simulink model "model"  (R2023b)
settings: Solver=FixedStepAuto  StartTime=0.0  StopTime=10.0  FixedStep=1e-3  RelTol=1e-3
InitFcn:
  | model_init
StopFcn:
  | animation;
values from neighbouring files (symbols this model uses):
  g = 9.81    [model_init.m]
  K = lqr(sys, Q, R)    [generate_controller.m]
  l = 1    [model_init.m]
  m = 0.5    [model_init.m]
  M = 1    [model_init.m]
  theta = out.simout.theta.Data    [animation.m]    (also in model_init.m = 0)
  theta_dot = 0    [model_init.m]
  x = out.simout.x.Data    [animation.m]    (also in model_init.m = 0)
  x_dot = 0    [model_init.m]
settings Model: Creator=zbyss  LastModifiedBy=zbyss

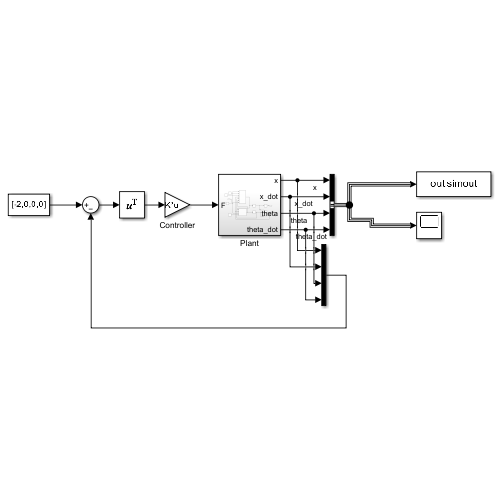
[thumbnail: Simulink's stored preview of the top-level diagram]
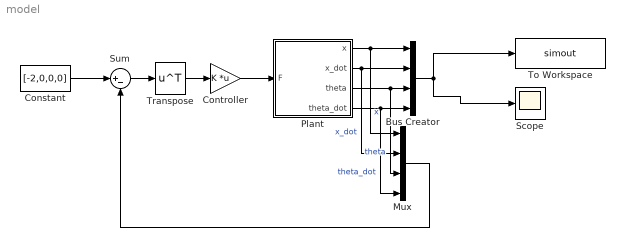
== system model ==
  Bus Creator : BusCreator  Inputs=4
  Constant : Constant  Value=[-2,0,0,0]
  Controller : Gain  Gain=K  Multiplication=Matrix(K*u)
  Mux : Mux
  Plant : Subsystem
  Scope : Scope
  Sum : Sum  Inputs=|+-
  To Workspace : ToWorkspace  VariableName=simout  SaveFormat=Timeseries  SampleTime=-1
  Transpose : Math  Operator=transpose
  wires:
  Plant/1(x) -> Bus Creator/1, Mux/1  "x"
  Plant/2(x_dot) -> Bus Creator/2, Mux/2  "x_dot"
  Plant/3(theta) -> Mux/3, Bus Creator/3  "theta"
  Plant/4(theta_dot) -> Mux/4, Bus Creator/4  "theta_dot"
  Bus Creator/1 -> To Workspace/1, Scope/1
  Controller/1 -> Plant/1(F)
  Transpose/1 -> Controller/1
  Sum/1 -> Transpose/1
  Mux/1 -> Sum/2
  Constant/1 -> Sum/1

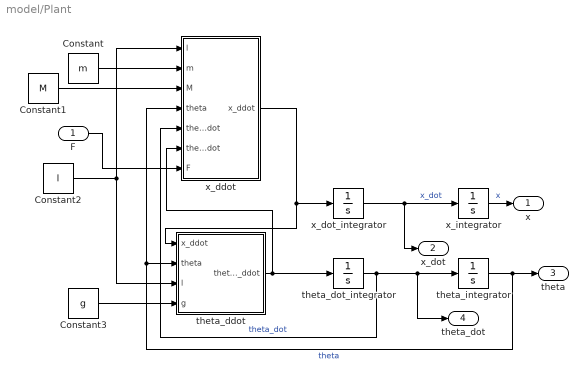
== system model/Plant ==
  F : Inport
  Constant : Constant  Value=m
  Constant1 : Constant  Value=M
  Constant2 : Constant  Value=l
  Constant3 : Constant  Value=g
  theta_ddot : Subsystem
  theta_dot_integrator : Integrator  InitialCondition=theta_dot
  theta_integrator : Integrator  InitialCondition=theta
  x_ddot : Subsystem
  x_dot_integrator : Integrator  InitialCondition=x_dot
  x_integrator : Integrator  InitialCondition=x
  x : Outport
  x_dot : Outport  Port=2
  theta : Outport  Port=3
  theta_dot : Outport  Port=4
  wires:
  Constant1/1 -> x_ddot/3(M)
  x_dot_integrator/1 -> x_integrator/1, x_dot/1  "x_dot"
  Constant2/1 -> theta_ddot/3(l), x_ddot/1(l)
  F/1 -> x_ddot/7(F)
  theta_dot_integrator/1 -> x_ddot/5(theta_dot), theta_integrator/1, theta_dot/1  "theta_dot"
  x_ddot/1(x_ddot) -> theta_ddot/1(x_ddot), x_dot_integrator/1
  theta_integrator/1 -> theta/1, theta_ddot/2(theta), x_ddot/4(theta)  "theta"
  theta_ddot/1(theta_ddot) -> x_ddot/6(theta_ddot), theta_dot_integrator/1
  x_integrator/1 -> x/1  "x"
  Constant3/1 -> theta_ddot/4(g)
  Constant/1 -> x_ddot/2(m)

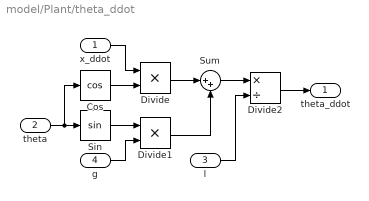
== system model/Plant/theta_ddot ==
  x_ddot : Inport
  theta : Inport  Port=2
  l : Inport  Port=3
  g : Inport  Port=4
  Cos : Trigonometry  Operator=cos
  Divide : Product  Inputs=**
  Divide1 : Product  Inputs=**
  Divide2 : Product  Inputs=*/
  Sin : Trigonometry
  Sum : Sum  Inputs=|++
  theta_ddot : Outport
  wires:
  theta/1 -> Cos/1, Sin/1
  x_ddot/1 -> Divide/1
  Cos/1 -> Divide/2
  Sin/1 -> Divide1/1
  g/1 -> Divide1/2
  Divide/1 -> Sum/1
  Divide1/1 -> Sum/2
  Sum/1 -> Divide2/1
  l/1 -> Divide2/2
  Divide2/1 -> theta_ddot/1

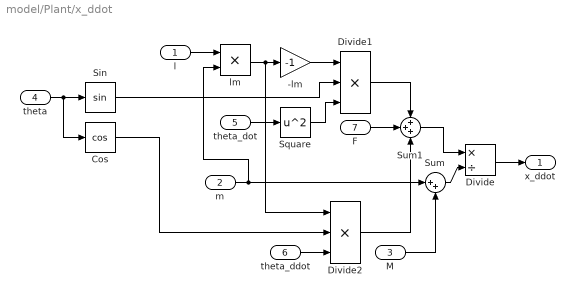
== system model/Plant/x_ddot ==
  l : Inport
  m : Inport  Port=2
  M : Inport  Port=3
  theta : Inport  Port=4
  theta_dot : Inport  Port=5
  theta_ddot : Inport  Port=6
  F : Inport  Port=7
  -lm : Gain  Gain=-1
  Cos : Trigonometry  Operator=cos
  Divide : Product  Inputs=*/
  Divide1 : Product  Inputs=***
  Divide2 : Product  Inputs=***
  Sin : Trigonometry
  Square : Math  Operator=square
  Sum : Sum  Inputs=|++
  Sum1 : Sum  Inputs=+++
  lm : Product  Inputs=**
  x_ddot : Outport
  wires:
  Divide/1 -> x_ddot/1
  Sum/1 -> Divide/2
  m/1 -> lm/2, Sum/1
  M/1 -> Sum/2
  l/1 -> lm/1
  lm/1 -> Divide2/1, -lm/1
  theta/1 -> Cos/1, Sin/1
  theta_dot/1 -> Square/1
  -lm/1 -> Divide1/1
  Sin/1 -> Divide1/2
  Square/1 -> Divide1/3
  Divide1/1 -> Sum1/1
  Sum1/1 -> Divide/1
  F/1 -> Sum1/2
  Divide2/1 -> Sum1/3
  theta_ddot/1 -> Divide2/3
  Cos/1 -> Divide2/2
